simulink model "SWC_FDC_type"  (R2021b)
settings: Solver=FixedStepDiscrete  StartTime=0.0  StopTime=10.0  FixedStep=0.001  RelTol=1e-3
values from neighbouring files (symbols this model uses):
  C_TASK_5MS_S = (	C_TICK_TIME_S      	)    [vcu_local_hdr.m]
  DID_VCUKey = uint16(0x0202)    [vcu_local_hdr.m]
  DID_XWD = uint16(513)    [vcu_local_hdr.m]
  DIDLen_APPPedalZP = uint16(3)    [vcu_local_hdr.m]
  DIDLen_APSFunConfig = uint16(16)    [vcu_local_hdr.m]
  DIDLen_AutoLock = uint16(1)    [vcu_local_hdr.m]
  DIDLen_AutoWipHSpdEN = uint16(1)    [vcu_local_hdr.m]
  DIDLen_DKCKey = uint16(8)    [vcu_local_hdr.m]
  DIDLen_DRLDis = uint16(1)    [vcu_local_hdr.m]
  DIDLen_DynoMode = uint16(1)    [vcu_local_hdr.m]
  DIDLen_FMHTimer = uint16(1)    [vcu_local_hdr.m]
  DIDLen_LFLowPresThre = uint16(1)    [vcu_local_hdr.m]
  DIDLen_LFSensorID = uint16(4)    [vcu_local_hdr.m]
  DIDLen_LRLowPresThre = uint16(1)    [vcu_local_hdr.m]
  DIDLen_LRSensorID = uint16(4)    [vcu_local_hdr.m]
  DIDLen_NVMPedalZP = uint16(3)    [vcu_local_hdr.m]
  DIDLen_RFLowPresThre = uint16(1)    [vcu_local_hdr.m]
  DIDLen_RFSensorID = uint16(4)    [vcu_local_hdr.m]
  DIDLen_RRLowPresThre = uint16(1)    [vcu_local_hdr.m]
  DIDLen_RRSensorID = uint16(4)    [vcu_local_hdr.m]
  DIDLen_SensorMode = uint16(1)    [vcu_local_hdr.m]
  DIDLen_TireSize = uint16(16)    [vcu_local_hdr.m]
  DIDLen_TPMSLearnSta = uint16(1)    [vcu_local_hdr.m]
  DIDLen_TurnLampFLThreCurr = uint16(1)    [vcu_local_hdr.m]
  DIDLen_TurnLampFRThreCurr = uint16(1)    [vcu_local_hdr.m]
  DIDLen_TurnLampRLThreCurr = uint16(1)    [vcu_local_hdr.m]
  DIDLen_TurnLampRRThreCurr = uint16(1)    [vcu_local_hdr.m]
  DIDLen_USSConfig = uint16(16)    [vcu_local_hdr.m]
  DIDLen_WhlPres = uint16(4)    [vcu_local_hdr.m]
  DIDLen_WhlSensorBattSta = uint16(1)    [vcu_local_hdr.m]
  DIDLen_WhlTmp = uint16(4)    [vcu_local_hdr.m]
  DIDLen_WipRLSCmdCutFilter = uint16(1)    [vcu_local_hdr.m]
  DIDLen_WipRLSCmdHoldFilter = uint16(1)    [vcu_local_hdr.m]
  DIDLen_XWDMode = uint16(1)    [vcu_local_hdr.m]
  DIDNum_APPPedalZP = uint16(0x0206)    [vcu_local_hdr.m]
  DIDNum_APSFunConfig = uint16(0x0903)    [vcu_local_hdr.m]
  DIDNum_AutoLock = uint16(0x0306)    [vcu_local_hdr.m]
  DIDNum_AutoWipHSpdEN = uint16(0x0308)    [vcu_local_hdr.m]
  DIDNum_DKCKey = uint16(0x0202)    [vcu_local_hdr.m]
  DIDNum_DRLDis = uint16(0x0307)    [vcu_local_hdr.m]
  DIDNum_DynoMode = uint16(0x0203)    [vcu_local_hdr.m]
  DIDNum_FMHTimer = uint16(0x0305)    [vcu_local_hdr.m]
  DIDNum_LFLowPresThre = uint16(0x0B08)    [vcu_local_hdr.m]
  DIDNum_LFSensorID = uint16(0x0B01)    [vcu_local_hdr.m]
  DIDNum_LRLowPresThre = uint16(0x0B0A)    [vcu_local_hdr.m]
  DIDNum_LRSensorID = uint16(0x0B03)    [vcu_local_hdr.m]
  DIDNum_NVMPedalZP = uint16(0x0207)    [vcu_local_hdr.m]
  DIDNum_RFLowPresThre = uint16(0x0B09)    [vcu_local_hdr.m]
  DIDNum_RFSensorID = uint16(0x0B02)    [vcu_local_hdr.m]
  DIDNum_RRLowPresThre = uint16(0x0B0B)    [vcu_local_hdr.m]
  DIDNum_RRSensorID = uint16(0x0B04)    [vcu_local_hdr.m]
  DIDNum_SensorMode = uint16(0x0B0C)    [vcu_local_hdr.m]
  DIDNum_TireSize = uint16(0x0902)    [vcu_local_hdr.m]
  DIDNum_TPMSLearnSta = uint16(0x0B0D)    [vcu_local_hdr.m]
  DIDNum_TurnLampFLThreCurr = uint16(0x0303)    [vcu_local_hdr.m]
  DIDNum_TurnLampFRThreCurr = uint16(0x0301)    [vcu_local_hdr.m]
  DIDNum_TurnLampRLThreCurr = uint16(0x0304)    [vcu_local_hdr.m]
  DIDNum_TurnLampRRThreCurr = uint16(0x0302)    [vcu_local_hdr.m]
  DIDNum_USSConfig = uint16(0x0901)    [vcu_local_hdr.m]
  DIDNum_WhlPres = uint16(0x0B05)    [vcu_local_hdr.m]
  DIDNum_WhlSensorBattSta = uint16(0x0B07)    [vcu_local_hdr.m]
  DIDNum_WhlTmp = uint16(0x0B06)    [vcu_local_hdr.m]
  DIDNum_WipRLSCmdCutFilter = uint16(0x030A)    [vcu_local_hdr.m]
  DIDNum_WipRLSCmdHoldFilter = uint16(0x0309)    [vcu_local_hdr.m]
  DIDNum_XWDMode = uint16(0x0201)    [vcu_local_hdr.m]
  DIDVCUKeyLength = uint16(8)    [vcu_local_hdr.m]
  DTC_10020B = Simulink.Parameter    [DTC_Constant_Definition.m]
  DTC_10020C = Simulink.Parameter    [DTC_Constant_Definition.m]
  DTC_10020D = Simulink.Parameter    [DTC_Constant_Definition.m]
  DTC_10020E = Simulink.Parameter    [DTC_Constant_Definition.m]
  DTC_100210 = Simulink.Parameter    [DTC_Constant_Definition.m]
  DTC_100211 = Simulink.Parameter    [DTC_Constant_Definition.m]
  DTC_100212 = Simulink.Parameter    [DTC_Constant_Definition.m]
  DTC_100213 = Simulink.Parameter    [DTC_Constant_Definition.m]
  DTC_100214 = Simulink.Parameter    [DTC_Constant_Definition.m]
  DTC_100215 = Simulink.Parameter    [DTC_Constant_Definition.m]
  DTC_100216 = Simulink.Parameter    [DTC_Constant_Definition.m]
  DTC_100217 = Simulink.Parameter    [DTC_Constant_Definition.m]
  DTC_100218 = Simulink.Parameter    [DTC_Constant_Definition.m]
  DTC_100219 = Simulink.Parameter    [DTC_Constant_Definition.m]
  DTC_10021A = Simulink.Parameter    [DTC_Constant_Definition.m]
  DTC_10021B = Simulink.Parameter    [DTC_Constant_Definition.m]
  DTC_10021C = Simulink.Parameter    [DTC_Constant_Definition.m]
  DTC_10021D = Simulink.Parameter    [DTC_Constant_Definition.m]
  DTC_10021E = Simulink.Parameter    [DTC_Constant_Definition.m]
  DTC_100220 = Simulink.Parameter    [DTC_Constant_Definition.m]
  DTC_100221 = Simulink.Parameter    [DTC_Constant_Definition.m]
  DTC_100223 = Simulink.Parameter    [DTC_Constant_Definition.m]
  DTC_100224 = Simulink.Parameter    [DTC_Constant_Definition.m]
  DTC_100225 = Simulink.Parameter    [DTC_Constant_Definition.m]
  DTC_100226 = Simulink.Parameter    [DTC_Constant_Definition.m]
  DTC_100227 = Simulink.Parameter    [DTC_Constant_Definition.m]
  DTC_100242 = Simulink.Parameter    [DTC_Constant_Definition.m]
  DTC_100243 = Simulink.Parameter    [DTC_Constant_Definition.m]
  DTC_100244 = Simulink.Parameter    [DTC_Constant_Definition.m]
  DTC_100247 = Simulink.Parameter    [DTC_Constant_Definition.m]
  DTC_100248 = Simulink.Parameter    [DTC_Constant_Definition.m]
  DTC_100249 = Simulink.Parameter    [DTC_Constant_Definition.m]
  DTC_100250 = Simulink.Parameter    [DTC_Constant_Definition.m]
  DTC_100251 = Simulink.Parameter    [DTC_Constant_Definition.m]
  DTC_100252 = Simulink.Parameter    [DTC_Constant_Definition.m]
  DTC_100A10 = Simulink.Parameter    [DTC_Constant_Definition.m]
  DTC_100A12 = Simulink.Parameter    [DTC_Constant_Definition.m]
  DTC_100A16 = Simulink.Parameter    [DTC_Constant_Definition.m]
  DTC_100A17 = Simulink.Parameter    [DTC_Constant_Definition.m]
  DTC_100A18 = Simulink.Parameter    [DTC_Constant_Definition.m]
  DTC_100A19 = Simulink.Parameter    [DTC_Constant_Definition.m]
  DTC_500B01 = Simulink.Parameter    [DTC_Constant_Definition.m]
  DTC_500B02 = Simulink.Parameter    [DTC_Constant_Definition.m]
  DTC_500B03 = Simulink.Parameter    [DTC_Constant_Definition.m]
  DTC_500B04 = Simulink.Parameter    [DTC_Constant_Definition.m]
  DTC_500B05 = Simulink.Parameter    [DTC_Constant_Definition.m]
  DTC_500B06 = Simulink.Parameter    [DTC_Constant_Definition.m]
  DTC_500B07 = Simulink.Parameter    [DTC_Constant_Definition.m]
  DTC_500B08 = Simulink.Parameter    [DTC_Constant_Definition.m]
  DTC_500B09 = Simulink.Parameter    [DTC_Constant_Definition.m]
  DTC_500B0A = Simulink.Parameter    [DTC_Constant_Definition.m]
  DTC_500B0B = Simulink.Parameter    [DTC_Constant_Definition.m]
  DTC_500B0C = Simulink.Parameter    [DTC_Constant_Definition.m]
  DTC_500B0D = Simulink.Parameter    [DTC_Constant_Definition.m]
  ... (+93 more)
undefined symbols (not defined in the file or in its folder): f32_ApsOutVehSpdSig, KHAL_CANBusOffDebounce_cnt, KHAL_CANBusOffDebounce_s, KHAL_DKCDecryptEnable_flg_ovrdflg, KHAL_DKCDecryptEnable_flg_ovrdval, KHAL_RandomNumberY1_enum, KHAL_RandomNumberY2_enum, KHAL_RandomNumberY_ovrdflg, KHAL_TPMSRESBUTT_flg_ovrdflg, KHAL_TPMSRESBUTT_flg_ovrdval, KINP_ReadVinCode_flg, KTQD_DefaultRegenMode_enum, R_DIDWriteCDD_CSOP_DIDSet_APPPedalZP, R_DIDWriteCDD_CSOP_DIDSet_APSFunConfig, R_DIDWriteCDD_CSOP_DIDSet_AutoLock, R_DIDWriteCDD_CSOP_DIDSet_AutoWipHSpdEN, R_DIDWriteCDD_CSOP_DIDSet_DKCKey, R_DIDWriteCDD_CSOP_DIDSet_DRLDis, R_DIDWriteCDD_CSOP_DIDSet_DynoMode, R_DIDWriteCDD_CSOP_DIDSet_FMHTimer, R_DIDWriteCDD_CSOP_DIDSet_LFLowPresThre, R_DIDWriteCDD_CSOP_DIDSet_LFSensorID, R_DIDWriteCDD_CSOP_DIDSet_LRLowPresThre, R_DIDWriteCDD_CSOP_DIDSet_LRSensorID, R_DIDWriteCDD_CSOP_DIDSet_NVMPedalZP, R_DIDWriteCDD_CSOP_DIDSet_RFLowPresThre, R_DIDWriteCDD_CSOP_DIDSet_RFSensorID, R_DIDWriteCDD_CSOP_DIDSet_RRLowPresThre, R_DIDWriteCDD_CSOP_DIDSet_RRSensorID, R_DIDWriteCDD_CSOP_DIDSet_SensorMode, R_DIDWriteCDD_CSOP_DIDSet_TireSize, R_DIDWriteCDD_CSOP_DIDSet_TPMSLearnSta, R_DIDWriteCDD_CSOP_DIDSet_TurnLampFLThreCurr, R_DIDWriteCDD_CSOP_DIDSet_TurnLampFRThreCurr, R_DIDWriteCDD_CSOP_DIDSet_TurnLampRLThreCurr, R_DIDWriteCDD_CSOP_DIDSet_TurnLampRRThreCurr, R_DIDWriteCDD_CSOP_DIDSet_USSConfig, R_DIDWriteCDD_CSOP_DIDSet_WhlPres, R_DIDWriteCDD_CSOP_DIDSet_WhlSensorBattSta, R_DIDWriteCDD_CSOP_DIDSet_WhlTmp, R_DIDWriteCDD_CSOP_DIDSet_WipRLSCmdCutFilter, R_DIDWriteCDD_CSOP_DIDSet_WipRLSCmdHoldFilter, R_DIDWriteCDD_CSOP_DIDSet_XWDMode, R_E2E_CAN3_VCU1_CSOP_Write_CAN3_VCU1, R_E2E_CAN3_VCU1_toNIDEC_CSOP_Write_CAN3_VCU1_toNIDEC ... (+128)
libraries: simulink x246, FVT_lib x139, hcu_lib x31, hdlsllib x11, app x1, halin x1, halout x1, matrix_library x1, inp x1, outp x1
(part 3 of 13)

== system SWC_FDC_type/run_SWC_FDC_Tx_1000ms_sys ==
  IRV_ms1000_CAN3_SG_GW_IVI6_toNIDEC_read : Inport
  function : TriggerPort  TriggerType=function-call  VariantControl=(inherit)  SampleTimeType=periodic  SampleTime=-1
  P_CAN3_GW_IVI6_toNIDEC_CAN3_SG_GW_IVI6_toNIDEC_write : Outport
  wires:
  IRV_ms1000_CAN3_SG_GW_IVI6_toNIDEC_read/1 -> P_CAN3_GW_IVI6_toNIDEC_CAN3_SG_GW_IVI6_toNIDEC_write/1

== system SWC_FDC_type/run_SWC_FDC_Tx_100ms_sys ==
  IRV_ms100_CAN1_SG_FD1_THCM1_read : Inport
  IRV_ms100_CAN3_SG_FD3_THCM1_read : Inport  Port=2
  function : TriggerPort  TriggerType=function-call  VariantControl=(inherit)  SampleTimeType=periodic  SampleTime=-1
  P_CAN1_FD1_THCM1_CAN1_SG_FD1_THCM1_write : Outport
  P_CAN3_FD3_THCM1_CAN3_SG_FD3_THCM1_write : Outport  Port=2
  wires:
  IRV_ms100_CAN1_SG_FD1_THCM1_read/1 -> P_CAN1_FD1_THCM1_CAN1_SG_FD1_THCM1_write/1
  IRV_ms100_CAN3_SG_FD3_THCM1_read/1 -> P_CAN3_FD3_THCM1_CAN3_SG_FD3_THCM1_write/1

== system SWC_FDC_type/run_SWC_FDC_Tx_10ms_sys ==
  IRV_ms10_CAN1_SG_FD1_APS3_read : Inport
  IRV_ms10_CAN1_SG_FD1_VCU2_read : Inport  Port=2
  IRV_ms10_CAN1_SG_FD1_VCU3_read : Inport  Port=3
  IRV_ms10_CAN1_SG_VMC_FCM1_read : Inport  Port=4
  IRV_ms10_CAN3_SG_FD3_VCU0_read : Inport  Port=5
  IRV_ms10_CAN3_SG_FD3_VCU2_read : Inport  Port=6
  IRV_ms10_CAN3_SG_FD3_VCU2_toNIDEC_read : Inport  Port=7
  IRV_ms10_CAN3_SG_FD3_VCU5_read : Inport  Port=8
  IRV_ms10_CAN3_SG_GW_ESC1_toNIDEC_read : Inport  Port=9
  IRV_ms10_CAN5_SG_FD5_Debug3_read : Inport  Port=10
  IRV_ms10_CAN6_SG_FD6_APS3_read : Inport  Port=11
  IRV_ms10_CAN6_SG_FD6_VCU2_read : Inport  Port=12
  IRV_f32_ApsOutVehSpdSig_read : Inport  Port=13
  IRV_u8_ApsOutGearPosnSig_read : Inport  Port=14
  IRV_u8_ApsOutSendChrgPlugSta_read : Inport  Port=15
  IRV_u8_ApsOutSetFrSensorOnCmd_read : Inport  Port=16
  IRV_u8_ApsOutSetFrSensorSwTOCmd_read : Inport  Port=17
  IRV_u8_ApsOutSetVehSpdTOCmd_read : Inport  Port=18
  function : TriggerPort  TriggerType=function-call  VariantControl=(inherit)  SampleTimeType=periodic  SampleTime=-1
  R_HALINCDD_CSOP_TPMS_GetRawData : FunctionCaller  FunctionPrototype=[u8_TPMSDataInSta,u8Array9_TPMSData] = R_HALINCDD_CSOP_TPMS_GetRawData()  OutputArgumentSpecifications=P_boolean, uint8([1;1;1;1;1;1;1;1;1])
  R_HALIN_APS_CSOP_ApsGetDist : FunctionCaller  FunctionPrototype=[u8Array8_PasInDist,u16Array4_ApsInDist] = R_HALIN_APS_CSOP_ApsGetDist()  OutputArgumentSpecifications=uint8([1;1;1;1;1;1;1;1]), uint16([1;1;1;1])
  R_HALIN_APS_CSOP_ApsGetDistLevel : FunctionCaller  FunctionPrototype=u8Array8_ApsInLevel = R_HALIN_APS_CSOP_ApsGetDistLevel()  OutputArgumentSpecifications=uint8([1;1;1;1;1;1;1;1])
  R_HALIN_APS_CSOP_ApsGetOtherStatus : FunctionCaller  FunctionPrototype=[u8_ApsInPASChime,u8_ApsInSensorLayout,u8_ApsInSysFailSta,u8_ApsInSysMode] = R_HALIN_APS_CSOP_ApsGetOtherStatus()  OutputArgumentSpecifications=uint8(1), uint8(1), uint8(1), uint8(1)
  R_HALIN_APS_CSOP_ApsGetUssSta : FunctionCaller  FunctionPrototype=u8Array12_ApsInUssSta = R_HALIN_APS_CSOP_ApsGetUssSta()  OutputArgumentSpecifications=uint8([1;1;1;1;1;1;1;1;1;1;1;1])
  R_HALOUT_APS_CSOP_ApsOutput : FunctionCaller  FunctionPrototype=R_HALOUT_APS_CSOP_ApsOutput(f32_ApsOutVehSpdSig,u8_ApsOutGearPosnSig,u8_ApsOutSetFrSensorOnCmd,u8_ApsOutSetVehSpdTOCmd,u8_ApsOutSetFrSensorSwTOCmd,u8_ApsOutSendChrgPlugSta)  InputArgumentSpecifications=single(1), uint8(1), uint8(1), uint8(1), uint8(1), uint8(1)
  P_CAN1_FD1_APS3_CAN1_SG_FD1_APS3_write : Outport
  P_CAN1_FD1_VCU2_CAN1_SG_FD1_VCU2_write : Outport  Port=2
  P_CAN1_FD1_VCU3_CAN1_SG_FD1_VCU3_write : Outport  Port=3
  P_CAN1_VMC_FCM1_CAN1_SG_VMC_FCM1_write : Outport  Port=4
  P_CAN3_FD3_VCU0_CAN3_SG_FD3_VCU0_write : Outport  Port=5
  P_CAN3_FD3_VCU2_CAN3_SG_FD3_VCU2_write : Outport  Port=6
  P_CAN3_FD3_VCU2_toNIDEC_CAN3_SG_FD3_VCU2_toNIDEC_write : Outport  Port=7
  P_CAN3_FD3_VCU5_CAN3_SG_FD3_VCU5_write : Outport  Port=8
  P_CAN3_GW_ESC1_toNIDEC_CAN3_SG_GW_ESC1_toNIDEC_write : Outport  Port=9
  P_CAN5_FD5_Debug3_CAN5_SG_FD5_Debug3_write : Outport  Port=10
  P_CAN6_FD6_APS3_CAN6_SG_FD6_APS3_write : Outport  Port=11
  P_CAN6_FD6_VCU2_CAN6_SG_FD6_VCU2_write : Outport  Port=12
  IRV_u16Array4_ApsInDist_write : Outport  Port=13  OutDataTypeStr=uint16  PortDimensions=4
  IRV_u8Array12_ApsInUssSta_write : Outport  Port=14  OutDataTypeStr=uint8  PortDimensions=12
  IRV_u8Array8_ApsInLevel_write : Outport  Port=15  OutDataTypeStr=uint8  PortDimensions=8
  IRV_u8Array8_PasInDist_write : Outport  Port=16  OutDataTypeStr=uint8  PortDimensions=8
  IRV_u8Array9_TPMSData_write : Outport  Port=17  OutDataTypeStr=uint8  PortDimensions=9
  IRV_u8_ApsInPASChime_write : Outport  Port=18  OutDataTypeStr=uint8  PortDimensions=1
  IRV_u8_ApsInSensorLayout_write : Outport  Port=19  OutDataTypeStr=uint8  PortDimensions=1
  IRV_u8_ApsInSysFailSta_write : Outport  Port=20  OutDataTypeStr=uint8  PortDimensions=1
  IRV_u8_ApsInSysMode_write : Outport  Port=21  OutDataTypeStr=uint8  PortDimensions=1
  IRV_u8_TPMSDataInSta_write : Outport  Port=22  OutDataTypeStr=uint8  PortDimensions=1
  wires:
  R_HALIN_APS_CSOP_ApsGetDist/1 -> IRV_u8Array8_PasInDist_write/1
  R_HALIN_APS_CSOP_ApsGetDist/2 -> IRV_u16Array4_ApsInDist_write/1
  R_HALIN_APS_CSOP_ApsGetDistLevel/1 -> IRV_u8Array8_ApsInLevel_write/1
  R_HALIN_APS_CSOP_ApsGetUssSta/1 -> IRV_u8Array12_ApsInUssSta_write/1
  IRV_f32_ApsOutVehSpdSig_read/1 -> R_HALOUT_APS_CSOP_ApsOutput/1
  IRV_u8_ApsOutGearPosnSig_read/1 -> R_HALOUT_APS_CSOP_ApsOutput/2
  IRV_u8_ApsOutSetFrSensorOnCmd_read/1 -> R_HALOUT_APS_CSOP_ApsOutput/3
  IRV_u8_ApsOutSetVehSpdTOCmd_read/1 -> R_HALOUT_APS_CSOP_ApsOutput/4
  IRV_u8_ApsOutSetFrSensorSwTOCmd_read/1 -> R_HALOUT_APS_CSOP_ApsOutput/5
  IRV_u8_ApsOutSendChrgPlugSta_read/1 -> R_HALOUT_APS_CSOP_ApsOutput/6
  R_HALIN_APS_CSOP_ApsGetOtherStatus/1 -> IRV_u8_ApsInPASChime_write/1
  R_HALIN_APS_CSOP_ApsGetOtherStatus/2 -> IRV_u8_ApsInSensorLayout_write/1
  R_HALIN_APS_CSOP_ApsGetOtherStatus/3 -> IRV_u8_ApsInSysFailSta_write/1
  R_HALIN_APS_CSOP_ApsGetOtherStatus/4 -> IRV_u8_ApsInSysMode_write/1
  R_HALINCDD_CSOP_TPMS_GetRawData/1 -> IRV_u8_TPMSDataInSta_write/1
  R_HALINCDD_CSOP_TPMS_GetRawData/2 -> IRV_u8Array9_TPMSData_write/1
  IRV_ms10_CAN1_SG_FD1_APS3_read/1 -> P_CAN1_FD1_APS3_CAN1_SG_FD1_APS3_write/1
  IRV_ms10_CAN1_SG_FD1_VCU2_read/1 -> P_CAN1_FD1_VCU2_CAN1_SG_FD1_VCU2_write/1
  IRV_ms10_CAN1_SG_FD1_VCU3_read/1 -> P_CAN1_FD1_VCU3_CAN1_SG_FD1_VCU3_write/1
  IRV_ms10_CAN1_SG_VMC_FCM1_read/1 -> P_CAN1_VMC_FCM1_CAN1_SG_VMC_FCM1_write/1
  IRV_ms10_CAN3_SG_FD3_VCU0_read/1 -> P_CAN3_FD3_VCU0_CAN3_SG_FD3_VCU0_write/1
  IRV_ms10_CAN3_SG_FD3_VCU2_toNIDEC_read/1 -> P_CAN3_FD3_VCU2_toNIDEC_CAN3_SG_FD3_VCU2_toNIDEC_write/1
  IRV_ms10_CAN3_SG_FD3_VCU5_read/1 -> P_CAN3_FD3_VCU5_CAN3_SG_FD3_VCU5_write/1
  IRV_ms10_CAN3_SG_GW_ESC1_toNIDEC_read/1 -> P_CAN3_GW_ESC1_toNIDEC_CAN3_SG_GW_ESC1_toNIDEC_write/1
  IRV_ms10_CAN5_SG_FD5_Debug3_read/1 -> P_CAN5_FD5_Debug3_CAN5_SG_FD5_Debug3_write/1
  IRV_ms10_CAN6_SG_FD6_APS3_read/1 -> P_CAN6_FD6_APS3_CAN6_SG_FD6_APS3_write/1
  IRV_ms10_CAN6_SG_FD6_VCU2_read/1 -> P_CAN6_FD6_VCU2_CAN6_SG_FD6_VCU2_write/1
  IRV_ms10_CAN3_SG_FD3_VCU2_read/1 -> P_CAN3_FD3_VCU2_CAN3_SG_FD3_VCU2_write/1

== system SWC_FDC_type/run_SWC_FDC_Tx_20ms_sys ==
  IRV_ms20_CAN1_SG_FD1_APS2_read : Inport
  IRV_ms20_CAN2_SG_FD2_C20_0_read : Inport  Port=2
  function : TriggerPort  TriggerType=function-call  VariantControl=(inherit)  SampleTimeType=periodic  SampleTime=-1
  P_CAN1_FD1_APS2_CAN1_SG_FD1_APS2_write : Outport
  P_CAN2_FD2_C20_0_CAN2_SG_FD2_C20_0_write : Outport  Port=2
  wires:
  IRV_ms20_CAN1_SG_FD1_APS2_read/1 -> P_CAN1_FD1_APS2_CAN1_SG_FD1_APS2_write/1
  IRV_ms20_CAN2_SG_FD2_C20_0_read/1 -> P_CAN2_FD2_C20_0_CAN2_SG_FD2_C20_0_write/1

== system SWC_FDC_type/run_SWC_FDC_Tx_5000ms_sys ==
  IRV_ms5000_CAN2_SG_FD2_Version_read : Inport
  function : TriggerPort  TriggerType=function-call  VariantControl=(inherit)  SampleTimeType=periodic  SampleTime=-1
  P_CAN2_FD2_Version_CAN2_SG_FD2_Version_write : Outport
  wires:
  IRV_ms5000_CAN2_SG_FD2_Version_read/1 -> P_CAN2_FD2_Version_CAN2_SG_FD2_Version_write/1

== system SWC_FDC_type/run_SWC_FDC_Tx_500ms_sys ==
  IRV_ms500_CAN1_SG_FD1_VMC2_read : Inport
  function : TriggerPort  TriggerType=function-call  VariantControl=(inherit)  SampleTimeType=periodic  SampleTime=-1
  P_CAN1_FD1_VMC2_CAN1_SG_FD1_VMC2_write : Outport
  wires:
  IRV_ms500_CAN1_SG_FD1_VMC2_read/1 -> P_CAN1_FD1_VMC2_CAN1_SG_FD1_VMC2_write/1

== system SWC_FDC_type/run_SWC_FDC_UDS_10ms_sys ==
  function : TriggerPort  TriggerType=function-call  VariantControl=(inherit)  SampleTimeType=periodic  SampleTime=-1
  R_HALINCDD_CSOP_UDS_Main : FunctionCaller  FunctionPrototype=R_HALINCDD_CSOP_UDS_Main()

== system SWC_FDC_type/P_WDGCDD/run_SWC_FDC_AppCallWDG_End_sys ==
  function : TriggerPort  TriggerType=function-call  IsSimulinkFunction=on  FunctionName=run_SWC_FDC_AppCallWDG_End  VariantControl=(inherit)

== system SWC_FDC_type/P_WDGCDD/run_SWC_FDC_AppCallWDG_StartUp_sys ==
  function : TriggerPort  TriggerType=function-call  IsSimulinkFunction=on  FunctionName=run_SWC_FDC_AppCallWDG_StartUp  VariantControl=(inherit)

== system SWC_FDC_type/P_WDGCDD/run_SWC_FDC_AppCallWDG_sys ==
  function : TriggerPort  TriggerType=function-call  IsSimulinkFunction=on  FunctionName=run_SWC_FDC_AppCallWDG  VariantControl=(inherit)

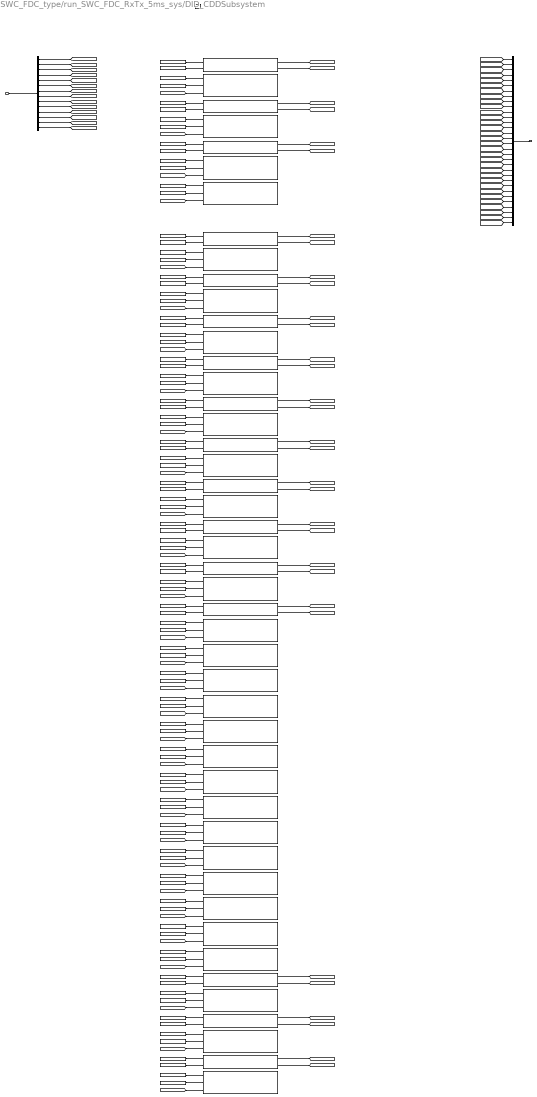
== system SWC_FDC_type/run_SWC_FDC_RxTx_5ms_sys/DID_CDDSubsystem ==
  BOUTP_DIDSetData_outputs : Inport
  trig_GetDID : TriggerPort  TriggerType=function-call  VariantControl=(inherit)  PortDimensions=1
  DIDLen : Constant  Value=DIDNum_XWDMode
  DIDLen1 : Constant  Value=DIDNum_XWDMode
  DIDLen10 : Constant  Value=DIDNum_TurnLampRRThreCurr
  DIDLen11 : Constant  Value=DIDNum_TurnLampFLThreCurr
  DIDLen12 : Constant  Value=DIDNum_TurnLampFLThreCurr
  DIDLen13 : Constant  Value=DIDNum_TurnLampRLThreCurr
  DIDLen14 : Constant  Value=DIDNum_TurnLampRLThreCurr
  DIDLen15 : Constant  Value=DIDNum_FMHTimer
  DIDLen16 : Constant  Value=DIDNum_FMHTimer
  DIDLen17 : Constant  Value=DIDNum_AutoLock
  DIDLen18 : Constant  Value=DIDNum_AutoLock
  DIDLen19 : Constant  Value=DIDNum_DRLDis
  DIDLen2 : Constant  Value=DIDNum_DKCKey
  DIDLen20 : Constant  Value=DIDNum_DRLDis
  DIDLen21 : Constant  Value=DIDNum_AutoWipHSpdEN
  DIDLen22 : Constant  Value=DIDNum_AutoWipHSpdEN
  DIDLen23 : Constant  Value=DIDNum_WipRLSCmdHoldFilter
  DIDLen24 : Constant  Value=DIDNum_WipRLSCmdHoldFilter
  DIDLen25 : Constant  Value=DIDNum_WipRLSCmdCutFilter
  DIDLen26 : Constant  Value=DIDNum_WipRLSCmdCutFilter
  DIDLen27 : Constant  Value=DIDNum_LFSensorID
  DIDLen28 : Constant  Value=DIDNum_RFSensorID
  DIDLen29 : Constant  Value=DIDNum_LRSensorID
  DIDLen3 : Constant  Value=DIDNum_DKCKey
  DIDLen30 : Constant  Value=DIDNum_RRSensorID
  DIDLen31 : Constant  Value=DIDNum_WhlPres
  DIDLen32 : Constant  Value=DIDNum_WhlTmp
  DIDLen33 : Constant  Value=DIDNum_WhlSensorBattSta
  DIDLen34 : Constant  Value=DIDNum_LFLowPresThre
  DIDLen35 : Constant  Value=DIDNum_RFLowPresThre
  DIDLen36 : Constant  Value=DIDNum_LRLowPresThre
  DIDLen37 : Constant  Value=DIDNum_RRLowPresThre
  DIDLen38 : Constant  Value=DIDNum_SensorMode
  DIDLen39 : Constant  Value=DIDNum_TPMSLearnSta
  DIDLen4 : Constant  Value=DIDNum_DynoMode
  DIDLen40 : Constant  Value=DIDNum_USSConfig
  DIDLen41 : Constant  Value=DIDNum_USSConfig
  DIDLen42 : Constant  Value=DIDNum_TireSize
  DIDLen43 : Constant  Value=DIDNum_TireSize
  DIDLen44 : Constant  Value=DIDNum_APSFunConfig
  DIDLen45 : Constant  Value=DIDNum_APSFunConfig
  DIDLen5 : Constant  Value=DIDNum_DynoMode
  DIDLen6 : Constant  Value=DIDNum_APPPedalZP
  DIDLen7 : Constant  Value=DIDNum_TurnLampFRThreCurr
  DIDLen8 : Constant  Value=DIDNum_TurnLampFRThreCurr
  DIDLen9 : Constant  Value=DIDNum_TurnLampRRThreCurr
  DIDNum : Constant  Value=DIDLen_XWDMode
  DIDNum1 : Constant  Value=DIDLen_XWDMode
  DIDNum10 : Constant  Value=DIDLen_TurnLampRRThreCurr
  DIDNum11 : Constant  Value=DIDLen_TurnLampFLThreCurr
  DIDNum12 : Constant  Value=DIDLen_TurnLampFLThreCurr
  DIDNum13 : Constant  Value=DIDLen_TurnLampRLThreCurr
  DIDNum14 : Constant  Value=DIDLen_TurnLampRLThreCurr
  DIDNum15 : Constant  Value=DIDLen_FMHTimer
  DIDNum16 : Constant  Value=DIDLen_FMHTimer
  DIDNum17 : Constant  Value=DIDLen_AutoLock
  DIDNum18 : Constant  Value=DIDLen_AutoLock
  DIDNum19 : Constant  Value=DIDLen_DRLDis
  DIDNum2 : Constant  Value=DIDLen_DKCKey
  DIDNum20 : Constant  Value=DIDLen_DRLDis
  DIDNum21 : Constant  Value=DIDLen_AutoWipHSpdEN
  DIDNum22 : Constant  Value=DIDLen_AutoWipHSpdEN
  DIDNum23 : Constant  Value=DIDLen_WipRLSCmdHoldFilter
  DIDNum24 : Constant  Value=DIDLen_WipRLSCmdHoldFilter
  DIDNum25 : Constant  Value=DIDLen_WipRLSCmdCutFilter
  DIDNum26 : Constant  Value=DIDLen_WipRLSCmdCutFilter
  DIDNum27 : Constant  Value=DIDLen_LFSensorID
  DIDNum28 : Constant  Value=DIDLen_RFSensorID
  DIDNum29 : Constant  Value=DIDLen_LRSensorID
  DIDNum3 : Constant  Value=DIDLen_DKCKey
  DIDNum30 : Constant  Value=DIDLen_RRSensorID
  DIDNum31 : Constant  Value=DIDLen_WhlPres
  DIDNum32 : Constant  Value=DIDLen_WhlTmp
  DIDNum33 : Constant  Value=DIDLen_WhlSensorBattSta
  DIDNum34 : Constant  Value=DIDLen_LFLowPresThre
  DIDNum35 : Constant  Value=DIDLen_RFLowPresThre
  DIDNum36 : Constant  Value=DIDLen_LRLowPresThre
  DIDNum37 : Constant  Value=DIDLen_RRLowPresThre
  DIDNum38 : Constant  Value=DIDLen_SensorMode
  DIDNum39 : Constant  Value=DIDLen_TPMSLearnSta
  DIDNum4 : Constant  Value=DIDLen_DynoMode
  DIDNum40 : Constant  Value=DIDLen_USSConfig
  DIDNum41 : Constant  Value=DIDLen_USSConfig
  DIDNum42 : Constant  Value=DIDLen_TireSize
  DIDNum43 : Constant  Value=DIDLen_TireSize
  DIDNum44 : Constant  Value=DIDLen_APSFunConfig
  DIDNum45 : Constant  Value=DIDLen_APSFunConfig
  DIDNum5 : Constant  Value=DIDLen_DynoMode
  DIDNum6 : Constant  Value=DIDLen_APPPedalZP
  DIDNum7 : Constant  Value=DIDLen_TurnLampFRThreCurr
  DIDNum8 : Constant  Value=DIDLen_TurnLampFRThreCurr
  DIDNum9 : Constant  Value=DIDLen_TurnLampRRThreCurr
  R_DIDReadCDD_CSOP_DIDGet_APSFunConfig : FunctionCaller  FunctionPrototype=[u8Array16_APSFunConfig,u8_DIDSta_APSFunConfig] = R_DIDReadCDD_CSOP_DIDGet_APSFunConfig(u16_DIDNum_APSFunConfig,u16_DIDLen_APSFunConfig)  InputArgumentSpecifications=uint16(1), uint16(1)  OutputArgumentSpecifications=uint8([1;1;1;1;1;1;1;1;1;1;1;1;1;1;1;1]), uint8(1)
  R_DIDReadCDD_CSOP_DIDGet_AutoLock : FunctionCaller  FunctionPrototype=[u8_AutoLock,u8_DIDSta_AutoLock] = R_DIDReadCDD_CSOP_DIDGet_AutoLock(u16_DIDNum_AutoLock,u16_DIDLen_AutoLock)  InputArgumentSpecifications=uint16(1), uint16(1)  OutputArgumentSpecifications=uint8(1), uint8(1)
  R_DIDReadCDD_CSOP_DIDGet_AutoWipHSpdEN : FunctionCaller  FunctionPrototype=[u8_AutoWipHSpdEN,u8_DIDSta_AutoWipHSpdEN] = R_DIDReadCDD_CSOP_DIDGet_AutoWipHSpdEN(u16_DIDNum_AutoWipHSpdEN,u16_DIDLen_AutoWipHSpdEN)  InputArgumentSpecifications=uint16(1), uint16(1)  OutputArgumentSpecifications=uint8(1), uint8(1)
  R_DIDReadCDD_CSOP_DIDGet_DKCKey : FunctionCaller  FunctionPrototype=[u8Array8_DKCKey,u8_DIDSta_DKCKey] = R_DIDReadCDD_CSOP_DIDGet_DKCKey(u16_DIDNum_DKCKey,u16_DIDLen_DKCKey)  InputArgumentSpecifications=uint16(1), uint16(1)  OutputArgumentSpecifications=uint8([1;1;1;1;1;1;1;1]), uint8(1)
  R_DIDReadCDD_CSOP_DIDGet_DRLDis : FunctionCaller  FunctionPrototype=[u8_DRLDis,u8_DIDSta_DRLDis] = R_DIDReadCDD_CSOP_DIDGet_DRLDis(u16_DIDNum_DRLDis,u16_DIDLen_DRLDis)  InputArgumentSpecifications=uint16(1), uint16(1)  OutputArgumentSpecifications=uint8(1), uint8(1)
  R_DIDReadCDD_CSOP_DIDGet_DynoMode : FunctionCaller  FunctionPrototype=[u8_DynoMode,u8_DIDSta_DynoMode] = R_DIDReadCDD_CSOP_DIDGet_DynoMode(u16_DIDNum_DynoMode,u16_DIDLen_DynoMode)  InputArgumentSpecifications=uint16(1), uint16(1)  OutputArgumentSpecifications=uint8(1), uint8(1)
  R_DIDReadCDD_CSOP_DIDGet_FMHTimer : FunctionCaller  FunctionPrototype=[u8_FMHTimer,u8_DIDSta_FMHTimer] = R_DIDReadCDD_CSOP_DIDGet_FMHTimer(u16_DIDNum_FMHTimer,u16_DIDLen_FMHTimer)  InputArgumentSpecifications=uint16(1), uint16(1)  OutputArgumentSpecifications=uint8(1), uint8(1)
  R_DIDReadCDD_CSOP_DIDGet_TireSize : FunctionCaller  FunctionPrototype=[u8Array16_TireSize,u8_DIDSta_TireSize] = R_DIDReadCDD_CSOP_DIDGet_TireSize(u16_DIDNum_TireSize,u16_DIDLen_TireSize)  InputArgumentSpecifications=uint16(1), uint16(1)  OutputArgumentSpecifications=uint8([1;1;1;1;1;1;1;1;1;1;1;1;1;1;1;1]), uint8(1)
  R_DIDReadCDD_CSOP_DIDGet_TurnLampFLThreCurr : FunctionCaller  FunctionPrototype=[u8_TurnLampFLThreCurr,u8_DIDSta_TurnLampFLThreCurr] = R_DIDReadCDD_CSOP_DIDGet_TurnLampFLThreCurr(u16_DIDNum_TurnLampFLThreCurr,u16_DIDLen_TurnLampFLThreCurr)  InputArgumentSpecifications=uint16(1), uint16(1)  OutputArgumentSpecifications=uint8(1), uint8(1)
  R_DIDReadCDD_CSOP_DIDGet_TurnLampFRThreCurr : FunctionCaller  FunctionPrototype=[u8_TurnLampFRThreCurr,u8_DIDSta_TurnLampFRThreCurr] = R_DIDReadCDD_CSOP_DIDGet_TurnLampFRThreCurr(u16_DIDNum_TurnLampFRThreCurr,u16_DIDLen_TurnLampFRThreCurr)  InputArgumentSpecifications=uint16(1), uint16(1)  OutputArgumentSpecifications=uint8(1), uint8(1)
  R_DIDReadCDD_CSOP_DIDGet_TurnLampRLThreCurr : FunctionCaller  FunctionPrototype=[u8_TurnLampRLThreCurr,u8_DIDSta_TurnLampRLThreCurr] = R_DIDReadCDD_CSOP_DIDGet_TurnLampRLThreCurr(u16_DIDNum_TurnLampRLThreCurr,u16_DIDLen_TurnLampRLThreCurr)  InputArgumentSpecifications=uint16(1), uint16(1)  OutputArgumentSpecifications=uint8(1), uint8(1)
  R_DIDReadCDD_CSOP_DIDGet_TurnLampRRThreCurr : FunctionCaller  FunctionPrototype=[u8_TurnLampRRThreCurr,u8_DIDSta_TurnLampRRThreCurr] = R_DIDReadCDD_CSOP_DIDGet_TurnLampRRThreCurr(u16_DIDNum_TurnLampRRThreCurr,u16_DIDLen_TurnLampRRThreCurr)  InputArgumentSpecifications=uint16(1), uint16(1)  OutputArgumentSpecifications=uint8(1), uint8(1)
  R_DIDReadCDD_CSOP_DIDGet_USSConfig : FunctionCaller  FunctionPrototype=[u8Array16_USSConfig,u8_DIDSta_USSConfig] = R_DIDReadCDD_CSOP_DIDGet_USSConfig(u16_DIDNum_USSConfig,u16_DIDLen_USSConfig)  InputArgumentSpecifications=uint16(1), uint16(1)  OutputArgumentSpecifications=uint8([1;1;1;1;1;1;1;1;1;1;1;1;1;1;1;1]), uint8(1)
  R_DIDReadCDD_CSOP_DIDGet_WipRLSCmdCutFilter : FunctionCaller  FunctionPrototype=[u8_WipRLSCmdCutFilter,u8_DIDSta_WipRLSCmdCutFilter] = R_DIDReadCDD_CSOP_DIDGet_WipRLSCmdCutFilter(u16_DIDNum_WipRLSCmdCutFilter,u16_DIDLen_WipRLSCmdCutFilter)  InputArgumentSpecifications=uint16(1), uint16(1)  OutputArgumentSpecifications=uint8(1), uint8(1)
  R_DIDReadCDD_CSOP_DIDGet_WipRLSCmdHoldFilter : FunctionCaller  FunctionPrototype=[u8_WipRLSCmdHoldFilter,u8_DIDSta_WipRLSCmdHoldFilter] = R_DIDReadCDD_CSOP_DIDGet_WipRLSCmdHoldFilter(u16_DIDNum_WipRLSCmdHoldFilter,u16_DIDLen_WipRLSCmdHoldFilter)  InputArgumentSpecifications=uint16(1), uint16(1)  OutputArgumentSpecifications=uint8(1), uint8(1)
  R_DIDReadCDD_CSOP_DIDGet_XWDMode : FunctionCaller  FunctionPrototype=[u8_XWDMode,u8_DIDSta_XWDMode] = R_DIDReadCDD_CSOP_DIDGet_XWDMode(u16_DIDNum_XWDMode,u16_DIDLen_XWDMode)  InputArgumentSpecifications=uint16(1), uint16(1)  OutputArgumentSpecifications=uint8(1), uint8(1)
  R_DIDWriteCDD_CSOP_DIDSet_APPPedalZP : FunctionCaller  FunctionPrototype=R_DIDWriteCDD_CSOP_DIDSet_APPPedalZP(u16_DIDNum_APPPedalZP,u16_DIDLen_APPPedalZP,u8Array3_APPPedalZP)  InputArgumentSpecifications=uint16(1), uint16(1), uint8([1;1;1])
  R_DIDWriteCDD_CSOP_DIDSet_APSFunConfig : FunctionCaller  FunctionPrototype=R_DIDWriteCDD_CSOP_DIDSet_APSFunConfig(u16_DIDNum_APSFunConfig,u16_DIDLen_APSFunConfig,u8Array16_APSFunConfig)  InputArgumentSpecifications=uint16(1), uint16(1), uint8([1;1;1;1;1;1;1;1;1;1;1;1;1;1;1;1])
  R_DIDWriteCDD_CSOP_DIDSet_AutoLock : FunctionCaller  FunctionPrototype=R_DIDWriteCDD_CSOP_DIDSet_AutoLock(u16_DIDNum_AutoLock,u16_DIDLen_AutoLock,u8_AutoLock)  InputArgumentSpecifications=uint16(1), uint16(1), uint8(1)
  R_DIDWriteCDD_CSOP_DIDSet_AutoWipHSpdEN : FunctionCaller  FunctionPrototype=R_DIDWriteCDD_CSOP_DIDSet_AutoWipHSpdEN(u16_DIDNum_AutoWipHSpdEN,u16_DIDLen_AutoWipHSpdEN,u8_AutoWipHSpdEN)  InputArgumentSpecifications=uint16(1), uint16(1), uint8(1)
  R_DIDWriteCDD_CSOP_DIDSet_DKCKey : FunctionCaller  FunctionPrototype=R_DIDWriteCDD_CSOP_DIDSet_DKCKey(u16_DIDNum_DKCKey,u16_DIDLen_DKCKey,u8Array8_DKCKey)  InputArgumentSpecifications=uint16(1), uint16(1), uint8([1;1;1;1;1;1;1;1])
  R_DIDWriteCDD_CSOP_DIDSet_DRLDis : FunctionCaller  FunctionPrototype=R_DIDWriteCDD_CSOP_DIDSet_DRLDis(u16_DIDNum_DRLDis,u16_DIDLen_DRLDis,u8_DRLDis)  InputArgumentSpecifications=uint16(1), uint16(1), uint8(1)
  R_DIDWriteCDD_CSOP_DIDSet_DynoMode : FunctionCaller  FunctionPrototype=R_DIDWriteCDD_CSOP_DIDSet_DynoMode(u16_DIDNum_DynoMode,u16_DIDLen_DynoMode,u8_DynoMode)  InputArgumentSpecifications=uint16(1), uint16(1), uint8(1)
  R_DIDWriteCDD_CSOP_DIDSet_FMHTimer : FunctionCaller  FunctionPrototype=R_DIDWriteCDD_CSOP_DIDSet_FMHTimer(u16_DIDNum_FMHTimer,u16_DIDLen_FMHTimer,u8_FMHTimer)  InputArgumentSpecifications=uint16(1), uint16(1), uint8(1)
  R_DIDWriteCDD_CSOP_DIDSet_LFLowPresThre : FunctionCaller  FunctionPrototype=R_DIDWriteCDD_CSOP_DIDSet_LFLowPresThre(u16_DIDNum_LFLowPresThre,u16_DIDLen_LFLowPresThre,u8_LFLowPresThre)  InputArgumentSpecifications=uint16(1), uint16(1), uint8(1)
  R_DIDWriteCDD_CSOP_DIDSet_LFSensorID : FunctionCaller  FunctionPrototype=R_DIDWriteCDD_CSOP_DIDSet_LFSensorID(u16_DIDNum_LFSensorID,u16_DIDLen_LFSensorID,u8Array4_LFSensorID)  InputArgumentSpecifications=uint16(1), uint16(1), uint8([1;1;1;1])
  R_DIDWriteCDD_CSOP_DIDSet_LRLowPresThre : FunctionCaller  FunctionPrototype=R_DIDWriteCDD_CSOP_DIDSet_LRLowPresThre(u16_DIDNum_LRLowPresThre,u16_DIDLen_LRLowPresThre,u8_LRLowPresThre)  InputArgumentSpecifications=uint16(1), uint16(1), uint8(1)
  R_DIDWriteCDD_CSOP_DIDSet_LRSensorID : FunctionCaller  FunctionPrototype=R_DIDWriteCDD_CSOP_DIDSet_LRSensorID(u16_DIDNum_LRSensorID,u16_DIDLen_LRSensorID,u8Array4_LRSensorID)  InputArgumentSpecifications=uint16(1), uint16(1), uint8([1;1;1;1])
  R_DIDWriteCDD_CSOP_DIDSet_RFLowPresThre : FunctionCaller  FunctionPrototype=R_DIDWriteCDD_CSOP_DIDSet_RFLowPresThre(u16_DIDNum_RFLowPresThre,u16_DIDLen_RFLowPresThre,u8_RFLowPresThre)  InputArgumentSpecifications=uint16(1), uint16(1), uint8(1)
  R_DIDWriteCDD_CSOP_DIDSet_RFSensorID : FunctionCaller  FunctionPrototype=R_DIDWriteCDD_CSOP_DIDSet_RFSensorID(u16_DIDNum_RFSensorID,u16_DIDLen_RFSensorID,u8Array4_RFSensorID)  InputArgumentSpecifications=uint16(1), uint16(1), uint8([1;1;1;1])
  R_DIDWriteCDD_CSOP_DIDSet_RRLowPresThre : FunctionCaller  FunctionPrototype=R_DIDWriteCDD_CSOP_DIDSet_RRLowPresThre(u16_DIDNum_RRLowPresThre,u16_DIDLen_RRLowPresThre,u8_RRLowPresThre)  InputArgumentSpecifications=uint16(1), uint16(1), uint8(1)
  R_DIDWriteCDD_CSOP_DIDSet_RRSensorID : FunctionCaller  FunctionPrototype=R_DIDWriteCDD_CSOP_DIDSet_RRSensorID(u16_DIDNum_RRSensorID,u16_DIDLen_RRSensorID,u8Array4_RRSensorID)  InputArgumentSpecifications=uint16(1), uint16(1), uint8([1;1;1;1])
  R_DIDWriteCDD_CSOP_DIDSet_SensorMode : FunctionCaller  FunctionPrototype=R_DIDWriteCDD_CSOP_DIDSet_SensorMode(u16_DIDNum_SensorMode,u16_DIDLen_SensorMode,u8_SensorMode)  InputArgumentSpecifications=uint16(1), uint16(1), uint8(1)
  R_DIDWriteCDD_CSOP_DIDSet_TPMSLearnSta : FunctionCaller  FunctionPrototype=R_DIDWriteCDD_CSOP_DIDSet_TPMSLearnSta(u16_DIDNum_TPMSLearnSta,u16_DIDLen_TPMSLearnSta,u8_TPMSLearnSta)  InputArgumentSpecifications=uint16(1), uint16(1), uint8(1)
  R_DIDWriteCDD_CSOP_DIDSet_TireSize : FunctionCaller  FunctionPrototype=R_DIDWriteCDD_CSOP_DIDSet_TireSize(u16_DIDNum_TireSize,u16_DIDLen_TireSize,u8Array16_TireSize)  InputArgumentSpecifications=uint16(1), uint16(1), uint8([1;1;1;1;1;1;1;1;1;1;1;1;1;1;1;1])
  R_DIDWriteCDD_CSOP_DIDSet_TurnLampFLThreCurr : FunctionCaller  FunctionPrototype=R_DIDWriteCDD_CSOP_DIDSet_TurnLampFLThreCurr(u16_DIDNum_TurnLampFLThreCurr,u16_DIDLen_TurnLampFLThreCurr,u8_TurnLampFLThreCurr)  InputArgumentSpecifications=uint16(1), uint16(1), uint8(1)
  R_DIDWriteCDD_CSOP_DIDSet_TurnLampFRThreCurr : FunctionCaller  FunctionPrototype=R_DIDWriteCDD_CSOP_DIDSet_TurnLampFRThreCurr(u16_DIDNum_TurnLampFRThreCurr,u16_DIDLen_TurnLampFRThreCurr,u8_TurnLampFRThreCurr)  InputArgumentSpecifications=uint16(1), uint16(1), uint8(1)
  R_DIDWriteCDD_CSOP_DIDSet_TurnLampRLThreCurr : FunctionCaller  FunctionPrototype=R_DIDWriteCDD_CSOP_DIDSet_TurnLampRLThreCurr(u16_DIDNum_TurnLampRLThreCurr,u16_DIDLen_TurnLampRLThreCurr,u8_TurnLampRLThreCurr)  InputArgumentSpecifications=uint16(1), uint16(1), uint8(1)
  R_DIDWriteCDD_CSOP_DIDSet_TurnLampRRThreCurr : FunctionCaller  FunctionPrototype=R_DIDWriteCDD_CSOP_DIDSet_TurnLampRRThreCurr(u16_DIDNum_TurnLampRRThreCurr,u16_DIDLen_TurnLampRRThreCurr,u8_TurnLampRRThreCurr)  InputArgumentSpecifications=uint16(1), uint16(1), uint8(1)
  R_DIDWriteCDD_CSOP_DIDSet_USSConfig : FunctionCaller  FunctionPrototype=R_DIDWriteCDD_CSOP_DIDSet_USSConfig(u16_DIDNum_USSConfig,u16_DIDLen_USSConfig,u8Array16_USSConfig)  InputArgumentSpecifications=uint16(1), uint16(1), uint8([1;1;1;1;1;1;1;1;1;1;1;1;1;1;1;1])
  R_DIDWriteCDD_CSOP_DIDSet_WhlPres : FunctionCaller  FunctionPrototype=R_DIDWriteCDD_CSOP_DIDSet_WhlPres(u16_DIDNum_WhlPres,u16_DIDLen_WhlPres,u8Array4_WhlPres)  InputArgumentSpecifications=uint16(1), uint16(1), uint8([1;1;1;1])
  R_DIDWriteCDD_CSOP_DIDSet_WhlSensorBattSta : FunctionCaller  FunctionPrototype=R_DIDWriteCDD_CSOP_DIDSet_WhlSensorBattSta(u16_DIDNum_WhlSensorBattSta,u16_DIDLen_WhlSensorBattSta,u8_WhlSensorBattSta)  InputArgumentSpecifications=uint16(1), uint16(1), uint8(1)
  R_DIDWriteCDD_CSOP_DIDSet_WhlTmp : FunctionCaller  FunctionPrototype=R_DIDWriteCDD_CSOP_DIDSet_WhlTmp(u16_DIDNum_WhlTmp,u16_DIDLen_WhlTmp,u8Array4_WhlTmp)  InputArgumentSpecifications=uint16(1), uint16(1), uint8([1;1;1;1])
  R_DIDWriteCDD_CSOP_DIDSet_WipRLSCmdCutFilter : FunctionCaller  FunctionPrototype=R_DIDWriteCDD_CSOP_DIDSet_WipRLSCmdCutFilter(u16_DIDNum_WipRLSCmdCutFilter,u16_DIDLen_WipRLSCmdCutFilter,u8_WipRLSCmdCutFilter)  InputArgumentSpecifications=uint16(1), uint16(1), uint8(1)
  R_DIDWriteCDD_CSOP_DIDSet_WipRLSCmdHoldFilter : FunctionCaller  FunctionPrototype=R_DIDWriteCDD_CSOP_DIDSet_WipRLSCmdHoldFilter(u16_DIDNum_WipRLSCmdHoldFilter,u16_DIDLen_WipRLSCmdHoldFilter,u8_WipRLSCmdHoldFilter)  InputArgumentSpecifications=uint16(1), uint16(1), uint8(1)
  R_DIDWriteCDD_CSOP_DIDSet_XWDMode : FunctionCaller  FunctionPrototype=R_DIDWriteCDD_CSOP_DIDSet_XWDMode(u16_DIDNum_XWDMode,u16_DIDLen_XWDMode,u8_XWDMode)  InputArgumentSpecifications=uint16(1), uint16(1), uint8(1)
  bus_Creator : BusCreator  Inputs=32
  bus_selector : BusSelector  OutputSignals=VHAL_DIDSetAPPPedalZP_raw8,VHAL_DIDSetLFSensorID_raw8,VHAL_DIDSetRFSensorID_raw8,VHAL_DIDSetLRSensorID_raw8,VHAL_DIDSetRRSensorID_raw8,VHAL_DIDSetWhlPres_raw8,VHAL_DIDSetWhlTmp_raw8,VHAL_DIDSetWhlSensorBattSta_raw8,VHAL_DIDSetLFLowPresThre_raw8,VHAL_DIDSetRFLowPresThre_raw8,VHAL_DIDSetLRLowPresThre_raw8,VHAL_DIDSetRRLowPresThre_raw8,VHAL_DIDSetSensorMode_raw8,VHAL_DIDSetTPMSLearnSta_raw8
  BHAL_DIDGetData_raw : Outport
  wires:
  bus_selector/1 -> [u8Array3_APPPedalZP]  "<VHAL_DIDSetAPPPedalZP_raw8>"
  bus_selector/2 -> [u8Array4_LFSensorID]  "<VHAL_DIDSetLFSensorID_raw8>"
  bus_selector/3 -> [u8Array4_RFSensorID]  "<VHAL_DIDSetRFSensorID_raw8>"
  bus_selector/4 -> [u8Array4_LRSensorID]  "<VHAL_DIDSetLRSensorID_raw8>"
  bus_selector/5 -> [u8Array4_RRSensorID]  "<VHAL_DIDSetRRSensorID_raw8>"
  bus_selector/6 -> [u8Array4_WhlPres]  "<VHAL_DIDSetWhlPres_raw8>"
  bus_selector/7 -> [u8Array4_WhlTmp]  "<VHAL_DIDSetWhlTmp_raw8>"
  bus_selector/8 -> [u8_WhlSensorBattSta]  "<VHAL_DIDSetWhlSensorBattSta_raw8>"
  bus_selector/9 -> [u8_LFLowPresThre]  "<VHAL_DIDSetLFLowPresThre_raw8>"
  bus_selector/10 -> [u8_RFLowPresThre]  "<VHAL_DIDSetRFLowPresThre_raw8>"
  bus_selector/11 -> [u8_LRLowPresThre]  "<VHAL_DIDSetLRLowPresThre_raw8>"
  bus_selector/12 -> [u8_RRLowPresThre]  "<VHAL_DIDSetRRLowPresThre_raw8>"
  bus_selector/13 -> [u8_SensorMode]  "<VHAL_DIDSetSensorMode_raw8>"
  bus_selector/14 -> [u8_TPMSLearnSta]  "<VHAL_DIDSetTPMSLearnSta_raw8>"
  BOUTP_DIDSetData_outputs/1 -> bus_selector/1
  [u8_DIDSta_XWDMode] -> bus_Creator/1  "u8_DIDSta_XWDMode"
  [u8_XWDMode] -> bus_Creator/2  "u8_XWDMode"
  [u8_DIDSta_DKCKey] -> bus_Creator/3  "u8_DIDSta_DKCKey"
  [u8Array8_DKCKey] -> bus_Creator/4  "u8Array8_DKCKey"
  [u8_DIDSta_DynoMode] -> bus_Creator/5  "u8_DIDSta_DynoMode"
  [u8_DynoMode] -> bus_Creator/6  "u8_DynoMode"
  [u8_DIDSta_TurnLampFRThreCurr] -> bus_Creator/7  "u8_DIDSta_TurnLampFRThreCurr"
  [u8_TurnLampFRThreCurr] -> bus_Creator/8  "u8_TurnLampFRThreCurr"
  [u8_DIDSta_TurnLampRRThreCurr] -> bus_Creator/9  "u8_DIDSta_TurnLampRRThreCurr"
  [u8_TurnLampRRThreCurr] -> bus_Creator/10  "u8_TurnLampRRThreCurr"
  [u8_DIDSta_TurnLampFLThreCurr] -> bus_Creator/11  "u8_DIDSta_TurnLampFLThreCurr"
  [u8_TurnLampFLThreCurr] -> bus_Creator/12  "u8_TurnLampFLThreCurr"
  [u8_DIDSta_TurnLampRLThreCurr] -> bus_Creator/13  "u8_DIDSta_TurnLampRLThreCurr"
  [u8_TurnLampRLThreCurr] -> bus_Creator/14  "u8_TurnLampRLThreCurr"
  [u8_DIDSta_FMHTimer] -> bus_Creator/15  "u8_DIDSta_FMHTimer"
  [u8_FMHTimer] -> bus_Creator/16  "u8_FMHTimer"
  [u8_DIDSta_AutoLock] -> bus_Creator/17  "u8_DIDSta_AutoLock"
  [u8_AutoLock] -> bus_Creator/18  "u8_AutoLock"
  [u8_DIDSta_DRLDis] -> bus_Creator/19  "u8_DIDSta_DRLDis"
  [u8_DRLDis] -> bus_Creator/20  "u8_DRLDis"
  [u8_DIDSta_AutoWipHSpdEN] -> bus_Creator/21  "u8_DIDSta_AutoWipHSpdEN"
  [u8_AutoWipHSpdEN] -> bus_Creator/22  "u8_AutoWipHSpdEN"
  [u8_DIDSta_WipRLSCmdHoldFilter] -> bus_Creator/23  "u8_DIDSta_WipRLSCmdHoldFilter"
  [u8_WipRLSCmdHoldFilter] -> bus_Creator/24  "u8_WipRLSCmdHoldFilter"
  [u8_DIDSta_WipRLSCmdCutFilter] -> bus_Creator/25  "u8_DIDSta_WipRLSCmdCutFilter"
  [u8_WipRLSCmdCutFilter] -> bus_Creator/26  "u8_WipRLSCmdCutFilter"
  [u8_DIDSta_USSConfig] -> bus_Creator/27  "u8_DIDSta_USSConfig"
  [u8Array16_USSConfig] -> bus_Creator/28  "u8Array16_USSConfig"
  [u8_DIDSta_TireSize] -> bus_Creator/29  "u8_DIDSta_TireSize"
  [u8Array16_TireSize] -> bus_Creator/30  "u8Array16_TireSize"
  [u8_DIDSta_APSFunConfig] -> bus_Creator/31  "u8_DIDSta_APSFunConfig"
  [u8Array16_APSFunConfig] -> bus_Creator/32  "u8Array16_APSFunConfig"
  bus_Creator/1 -> BHAL_DIDGetData_raw/1
  DIDLen/1 -> R_DIDReadCDD_CSOP_DIDGet_XWDMode/1
  DIDNum/1 -> R_DIDReadCDD_CSOP_DIDGet_XWDMode/2
  R_DIDReadCDD_CSOP_DIDGet_XWDMode/1 -> [u8_XWDMode]
  R_DIDReadCDD_CSOP_DIDGet_XWDMode/2 -> [u8_DIDSta_XWDMode]
  DIDLen1/1 -> R_DIDWriteCDD_CSOP_DIDSet_XWDMode/1
  DIDNum1/1 -> R_DIDWriteCDD_CSOP_DIDSet_XWDMode/2
  [u8_XWDMode] -> R_DIDWriteCDD_CSOP_DIDSet_XWDMode/3
  DIDLen2/1 -> R_DIDReadCDD_CSOP_DIDGet_DKCKey/1
  DIDNum2/1 -> R_DIDReadCDD_CSOP_DIDGet_DKCKey/2
  R_DIDReadCDD_CSOP_DIDGet_DKCKey/1 -> [u8Array8_DKCKey]
  R_DIDReadCDD_CSOP_DIDGet_DKCKey/2 -> [u8_DIDSta_DKCKey]
  DIDLen3/1 -> R_DIDWriteCDD_CSOP_DIDSet_DKCKey/1
  DIDNum3/1 -> R_DIDWriteCDD_CSOP_DIDSet_DKCKey/2
  [u8Array8_DKCKey] -> R_DIDWriteCDD_CSOP_DIDSet_DKCKey/3
  DIDLen4/1 -> R_DIDReadCDD_CSOP_DIDGet_DynoMode/1
  DIDNum4/1 -> R_DIDReadCDD_CSOP_DIDGet_DynoMode/2
  R_DIDReadCDD_CSOP_DIDGet_DynoMode/1 -> [u8_DynoMode]
  R_DIDReadCDD_CSOP_DIDGet_DynoMode/2 -> [u8_DIDSta_DynoMode]
  DIDLen5/1 -> R_DIDWriteCDD_CSOP_DIDSet_DynoMode/1
  DIDNum5/1 -> R_DIDWriteCDD_CSOP_DIDSet_DynoMode/2
  [u8_DynoMode] -> R_DIDWriteCDD_CSOP_DIDSet_DynoMode/3
  DIDLen6/1 -> R_DIDWriteCDD_CSOP_DIDSet_APPPedalZP/1
  DIDNum6/1 -> R_DIDWriteCDD_CSOP_DIDSet_APPPedalZP/2
  [u8Array3_APPPedalZP] -> R_DIDWriteCDD_CSOP_DIDSet_APPPedalZP/3
  DIDLen7/1 -> R_DIDReadCDD_CSOP_DIDGet_TurnLampFRThreCurr/1
  DIDNum7/1 -> R_DIDReadCDD_CSOP_DIDGet_TurnLampFRThreCurr/2
  R_DIDReadCDD_CSOP_DIDGet_TurnLampFRThreCurr/1 -> [u8_TurnLampFRThreCurr]
  R_DIDReadCDD_CSOP_DIDGet_TurnLampFRThreCurr/2 -> [u8_DIDSta_TurnLampFRThreCurr]
  DIDLen8/1 -> R_DIDWriteCDD_CSOP_DIDSet_TurnLampFRThreCurr/1
  DIDNum8/1 -> R_DIDWriteCDD_CSOP_DIDSet_TurnLampFRThreCurr/2
  [u8_TurnLampFRThreCurr] -> R_DIDWriteCDD_CSOP_DIDSet_TurnLampFRThreCurr/3
  DIDLen9/1 -> R_DIDReadCDD_CSOP_DIDGet_TurnLampRRThreCurr/1
  DIDNum9/1 -> R_DIDReadCDD_CSOP_DIDGet_TurnLampRRThreCurr/2
  R_DIDReadCDD_CSOP_DIDGet_TurnLampRRThreCurr/1 -> [u8_TurnLampRRThreCurr]
  R_DIDReadCDD_CSOP_DIDGet_TurnLampRRThreCurr/2 -> [u8_DIDSta_TurnLampRRThreCurr]
  DIDLen10/1 -> R_DIDWriteCDD_CSOP_DIDSet_TurnLampRRThreCurr/1
  DIDNum10/1 -> R_DIDWriteCDD_CSOP_DIDSet_TurnLampRRThreCurr/2
  [u8_TurnLampRRThreCurr] -> R_DIDWriteCDD_CSOP_DIDSet_TurnLampRRThreCurr/3
  DIDLen11/1 -> R_DIDReadCDD_CSOP_DIDGet_TurnLampFLThreCurr/1
  DIDNum11/1 -> R_DIDReadCDD_CSOP_DIDGet_TurnLampFLThreCurr/2
  R_DIDReadCDD_CSOP_DIDGet_TurnLampFLThreCurr/1 -> [u8_TurnLampFLThreCurr]
  R_DIDReadCDD_CSOP_DIDGet_TurnLampFLThreCurr/2 -> [u8_DIDSta_TurnLampFLThreCurr]
  DIDLen12/1 -> R_DIDWriteCDD_CSOP_DIDSet_TurnLampFLThreCurr/1
  DIDNum12/1 -> R_DIDWriteCDD_CSOP_DIDSet_TurnLampFLThreCurr/2
  [u8_TurnLampFLThreCurr] -> R_DIDWriteCDD_CSOP_DIDSet_TurnLampFLThreCurr/3
  DIDLen13/1 -> R_DIDReadCDD_CSOP_DIDGet_TurnLampRLThreCurr/1
  DIDNum13/1 -> R_DIDReadCDD_CSOP_DIDGet_TurnLampRLThreCurr/2
  R_DIDReadCDD_CSOP_DIDGet_TurnLampRLThreCurr/1 -> [u8_TurnLampRLThreCurr]
  R_DIDReadCDD_CSOP_DIDGet_TurnLampRLThreCurr/2 -> [u8_DIDSta_TurnLampRLThreCurr]
  DIDLen14/1 -> R_DIDWriteCDD_CSOP_DIDSet_TurnLampRLThreCurr/1
  DIDNum14/1 -> R_DIDWriteCDD_CSOP_DIDSet_TurnLampRLThreCurr/2
  [u8_TurnLampRLThreCurr] -> R_DIDWriteCDD_CSOP_DIDSet_TurnLampRLThreCurr/3
  DIDLen15/1 -> R_DIDReadCDD_CSOP_DIDGet_FMHTimer/1
  DIDNum15/1 -> R_DIDReadCDD_CSOP_DIDGet_FMHTimer/2
  R_DIDReadCDD_CSOP_DIDGet_FMHTimer/1 -> [u8_FMHTimer]
  R_DIDReadCDD_CSOP_DIDGet_FMHTimer/2 -> [u8_DIDSta_FMHTimer]
  DIDLen16/1 -> R_DIDWriteCDD_CSOP_DIDSet_FMHTimer/1
  DIDNum16/1 -> R_DIDWriteCDD_CSOP_DIDSet_FMHTimer/2
  [u8_FMHTimer] -> R_DIDWriteCDD_CSOP_DIDSet_FMHTimer/3
  DIDLen17/1 -> R_DIDReadCDD_CSOP_DIDGet_AutoLock/1
  DIDNum17/1 -> R_DIDReadCDD_CSOP_DIDGet_AutoLock/2
  R_DIDReadCDD_CSOP_DIDGet_AutoLock/1 -> [u8_AutoLock]
  R_DIDReadCDD_CSOP_DIDGet_AutoLock/2 -> [u8_DIDSta_AutoLock]
  DIDLen18/1 -> R_DIDWriteCDD_CSOP_DIDSet_AutoLock/1
  DIDNum18/1 -> R_DIDWriteCDD_CSOP_DIDSet_AutoLock/2
  [u8_AutoLock] -> R_DIDWriteCDD_CSOP_DIDSet_AutoLock/3
  DIDLen19/1 -> R_DIDReadCDD_CSOP_DIDGet_DRLDis/1
  DIDNum19/1 -> R_DIDReadCDD_CSOP_DIDGet_DRLDis/2
  R_DIDReadCDD_CSOP_DIDGet_DRLDis/1 -> [u8_DRLDis]
  R_DIDReadCDD_CSOP_DIDGet_DRLDis/2 -> [u8_DIDSta_DRLDis]
  DIDLen20/1 -> R_DIDWriteCDD_CSOP_DIDSet_DRLDis/1
  DIDNum20/1 -> R_DIDWriteCDD_CSOP_DIDSet_DRLDis/2
  [u8_DRLDis] -> R_DIDWriteCDD_CSOP_DIDSet_DRLDis/3
  DIDLen21/1 -> R_DIDReadCDD_CSOP_DIDGet_AutoWipHSpdEN/1
  DIDNum21/1 -> R_DIDReadCDD_CSOP_DIDGet_AutoWipHSpdEN/2
  R_DIDReadCDD_CSOP_DIDGet_AutoWipHSpdEN/1 -> [u8_AutoWipHSpdEN]
  R_DIDReadCDD_CSOP_DIDGet_AutoWipHSpdEN/2 -> [u8_DIDSta_AutoWipHSpdEN]
  DIDLen22/1 -> R_DIDWriteCDD_CSOP_DIDSet_AutoWipHSpdEN/1
  DIDNum22/1 -> R_DIDWriteCDD_CSOP_DIDSet_AutoWipHSpdEN/2
  [u8_AutoWipHSpdEN] -> R_DIDWriteCDD_CSOP_DIDSet_AutoWipHSpdEN/3
  DIDLen23/1 -> R_DIDReadCDD_CSOP_DIDGet_WipRLSCmdHoldFilter/1
  DIDNum23/1 -> R_DIDReadCDD_CSOP_DIDGet_WipRLSCmdHoldFilter/2
  R_DIDReadCDD_CSOP_DIDGet_WipRLSCmdHoldFilter/1 -> [u8_WipRLSCmdHoldFilter]
  R_DIDReadCDD_CSOP_DIDGet_WipRLSCmdHoldFilter/2 -> [u8_DIDSta_WipRLSCmdHoldFilter]
  DIDLen24/1 -> R_DIDWriteCDD_CSOP_DIDSet_WipRLSCmdHoldFilter/1
  DIDNum24/1 -> R_DIDWriteCDD_CSOP_DIDSet_WipRLSCmdHoldFilter/2
  [u8_WipRLSCmdHoldFilter] -> R_DIDWriteCDD_CSOP_DIDSet_WipRLSCmdHoldFilter/3
  DIDLen25/1 -> R_DIDReadCDD_CSOP_DIDGet_WipRLSCmdCutFilter/1
  DIDNum25/1 -> R_DIDReadCDD_CSOP_DIDGet_WipRLSCmdCutFilter/2
  R_DIDReadCDD_CSOP_DIDGet_WipRLSCmdCutFilter/1 -> [u8_WipRLSCmdCutFilter]
  R_DIDReadCDD_CSOP_DIDGet_WipRLSCmdCutFilter/2 -> [u8_DIDSta_WipRLSCmdCutFilter]
  DIDLen26/1 -> R_DIDWriteCDD_CSOP_DIDSet_WipRLSCmdCutFilter/1
  DIDNum26/1 -> R_DIDWriteCDD_CSOP_DIDSet_WipRLSCmdCutFilter/2
  [u8_WipRLSCmdCutFilter] -> R_DIDWriteCDD_CSOP_DIDSet_WipRLSCmdCutFilter/3
  DIDLen27/1 -> R_DIDWriteCDD_CSOP_DIDSet_LFSensorID/1
  DIDNum27/1 -> R_DIDWriteCDD_CSOP_DIDSet_LFSensorID/2
  [u8Array4_LFSensorID] -> R_DIDWriteCDD_CSOP_DIDSet_LFSensorID/3
  DIDLen28/1 -> R_DIDWriteCDD_CSOP_DIDSet_RFSensorID/1
  DIDNum28/1 -> R_DIDWriteCDD_CSOP_DIDSet_RFSensorID/2
  [u8Array4_RFSensorID] -> R_DIDWriteCDD_CSOP_DIDSet_RFSensorID/3
  DIDLen29/1 -> R_DIDWriteCDD_CSOP_DIDSet_LRSensorID/1
  DIDNum29/1 -> R_DIDWriteCDD_CSOP_DIDSet_LRSensorID/2
  [u8Array4_LRSensorID] -> R_DIDWriteCDD_CSOP_DIDSet_LRSensorID/3
  DIDLen30/1 -> R_DIDWriteCDD_CSOP_DIDSet_RRSensorID/1
  DIDNum30/1 -> R_DIDWriteCDD_CSOP_DIDSet_RRSensorID/2
  [u8Array4_RRSensorID] -> R_DIDWriteCDD_CSOP_DIDSet_RRSensorID/3
  DIDLen31/1 -> R_DIDWriteCDD_CSOP_DIDSet_WhlPres/1
  DIDNum31/1 -> R_DIDWriteCDD_CSOP_DIDSet_WhlPres/2
  [u8Array4_WhlPres] -> R_DIDWriteCDD_CSOP_DIDSet_WhlPres/3
  DIDLen32/1 -> R_DIDWriteCDD_CSOP_DIDSet_WhlTmp/1
  DIDNum32/1 -> R_DIDWriteCDD_CSOP_DIDSet_WhlTmp/2
  [u8Array4_WhlTmp] -> R_DIDWriteCDD_CSOP_DIDSet_WhlTmp/3
  DIDLen33/1 -> R_DIDWriteCDD_CSOP_DIDSet_WhlSensorBattSta/1
  DIDNum33/1 -> R_DIDWriteCDD_CSOP_DIDSet_WhlSensorBattSta/2
  [u8_WhlSensorBattSta] -> R_DIDWriteCDD_CSOP_DIDSet_WhlSensorBattSta/3
  DIDLen34/1 -> R_DIDWriteCDD_CSOP_DIDSet_LFLowPresThre/1
  DIDNum34/1 -> R_DIDWriteCDD_CSOP_DIDSet_LFLowPresThre/2
  [u8_LFLowPresThre] -> R_DIDWriteCDD_CSOP_DIDSet_LFLowPresThre/3
  DIDLen35/1 -> R_DIDWriteCDD_CSOP_DIDSet_RFLowPresThre/1
  DIDNum35/1 -> R_DIDWriteCDD_CSOP_DIDSet_RFLowPresThre/2
  [u8_RFLowPresThre] -> R_DIDWriteCDD_CSOP_DIDSet_RFLowPresThre/3
  DIDLen36/1 -> R_DIDWriteCDD_CSOP_DIDSet_LRLowPresThre/1
  DIDNum36/1 -> R_DIDWriteCDD_CSOP_DIDSet_LRLowPresThre/2
  [u8_LRLowPresThre] -> R_DIDWriteCDD_CSOP_DIDSet_LRLowPresThre/3
  DIDLen37/1 -> R_DIDWriteCDD_CSOP_DIDSet_RRLowPresThre/1
  DIDNum37/1 -> R_DIDWriteCDD_CSOP_DIDSet_RRLowPresThre/2
  [u8_RRLowPresThre] -> R_DIDWriteCDD_CSOP_DIDSet_RRLowPresThre/3
  DIDLen38/1 -> R_DIDWriteCDD_CSOP_DIDSet_SensorMode/1
  DIDNum38/1 -> R_DIDWriteCDD_CSOP_DIDSet_SensorMode/2
  [u8_SensorMode] -> R_DIDWriteCDD_CSOP_DIDSet_SensorMode/3
  DIDLen39/1 -> R_DIDWriteCDD_CSOP_DIDSet_TPMSLearnSta/1
  DIDNum39/1 -> R_DIDWriteCDD_CSOP_DIDSet_TPMSLearnSta/2
  [u8_TPMSLearnSta] -> R_DIDWriteCDD_CSOP_DIDSet_TPMSLearnSta/3
  DIDLen40/1 -> R_DIDReadCDD_CSOP_DIDGet_USSConfig/1
  DIDNum40/1 -> R_DIDReadCDD_CSOP_DIDGet_USSConfig/2
  R_DIDReadCDD_CSOP_DIDGet_USSConfig/1 -> [u8Array16_USSConfig]
  R_DIDReadCDD_CSOP_DIDGet_USSConfig/2 -> [u8_DIDSta_USSConfig]
  DIDLen41/1 -> R_DIDWriteCDD_CSOP_DIDSet_USSConfig/1
  DIDNum41/1 -> R_DIDWriteCDD_CSOP_DIDSet_USSConfig/2
  [u8Array16_USSConfig] -> R_DIDWriteCDD_CSOP_DIDSet_USSConfig/3
  DIDLen42/1 -> R_DIDReadCDD_CSOP_DIDGet_TireSize/1
  DIDNum42/1 -> R_DIDReadCDD_CSOP_DIDGet_TireSize/2
  R_DIDReadCDD_CSOP_DIDGet_TireSize/1 -> [u8Array16_TireSize]
  R_DIDReadCDD_CSOP_DIDGet_TireSize/2 -> [u8_DIDSta_TireSize]
  DIDLen43/1 -> R_DIDWriteCDD_CSOP_DIDSet_TireSize/1
  DIDNum43/1 -> R_DIDWriteCDD_CSOP_DIDSet_TireSize/2
  [u8Array16_TireSize] -> R_DIDWriteCDD_CSOP_DIDSet_TireSize/3
  DIDLen44/1 -> R_DIDReadCDD_CSOP_DIDGet_APSFunConfig/1
  DIDNum44/1 -> R_DIDReadCDD_CSOP_DIDGet_APSFunConfig/2
  R_DIDReadCDD_CSOP_DIDGet_APSFunConfig/1 -> [u8Array16_APSFunConfig]
  R_DIDReadCDD_CSOP_DIDGet_APSFunConfig/2 -> [u8_DIDSta_APSFunConfig]
  DIDLen45/1 -> R_DIDWriteCDD_CSOP_DIDSet_APSFunConfig/1
  DIDNum45/1 -> R_DIDWriteCDD_CSOP_DIDSet_APSFunConfig/2
  [u8Array16_APSFunConfig] -> R_DIDWriteCDD_CSOP_DIDSet_APSFunConfig/3

== system SWC_FDC_type/run_SWC_FDC_RxTx_5ms_sys/Function-Call Subsystem ==
  u8Array256_NvmReadArray : Inport
  function : TriggerPort  TriggerType=function-call  VariantControl=(inherit)
  u8Array256_NvmReadArrayInit : Outport
  wires:
  u8Array256_NvmReadArray/1 -> u8Array256_NvmReadArrayInit/1
